simulink model "FMTM"  (R2022b)
settings: Solver=FixedStepAuto  StartTime=0.0  StopTime=10.0  FixedStep=1  RelTol=1e-3
libraries: simulink x34
settings Model: Creator=sadamu  LastModifiedBy=yuzehong
settings OptimizationCC: DefaultParameterBehavior=Inlined  BufferReuse=off  GlobalBufferReuse=off  ExpressionFolding=off  EnableMemcpy=off  PassReuseOutputArgsAs=Individual arguments  NoFixptDivByZeroProtection=on  EfficientFloat2IntCast=on  OptimizeDataStoreBuffers=off  BusAssignmentInplaceUpdate=off  OptimizationLevel=level0  EfficientTunableParamExpr=on
settings DebuggingCC: ParameterTunabilityLossMsg=error  AllowSymbolicDim=off
settings SFSimCC: MATLABDynamicMemAlloc=off
settings RTWCC: Description=Embedded Coder  SystemTargetFile=ert.tlc  GenCodeOnly=on  TemplateMakefile=ert_default_tmf
settings CodeAppCC: GenerateComments=off  IgnoreCustomStorageClasses=off  OperatorAnnotations=on  SimulinkDataObjDesc=on  SFDataObjDesc=on  SimulinkBlockComments=off
settings ERTTargetCC: TargetLangStandard=C99 (ISO)  GenerateSampleERTMain=on  CodeInterfacePackaging=Reusable function  InlinedParameterPlacement=NonHierarchical  ERTCustomFileTemplate=example_file_process.tlc
settings ConfigComp: CovMetricSettings=dcmwe  DVMaxProcessTime=3600  DVTestSuiteOptimization=Auto  DVDetectOutOfBounds=on  DVModelReferenceHarness=on

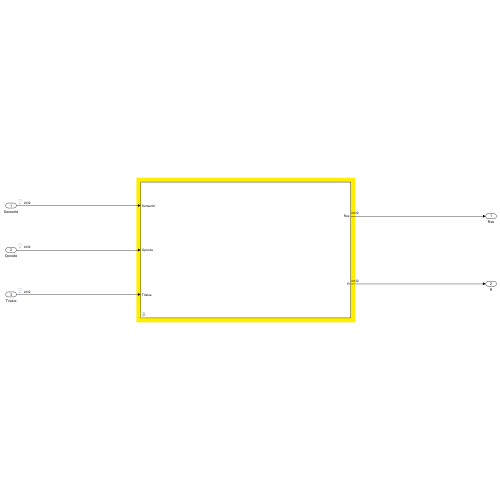
[thumbnail: Simulink's stored preview of the top-level diagram]
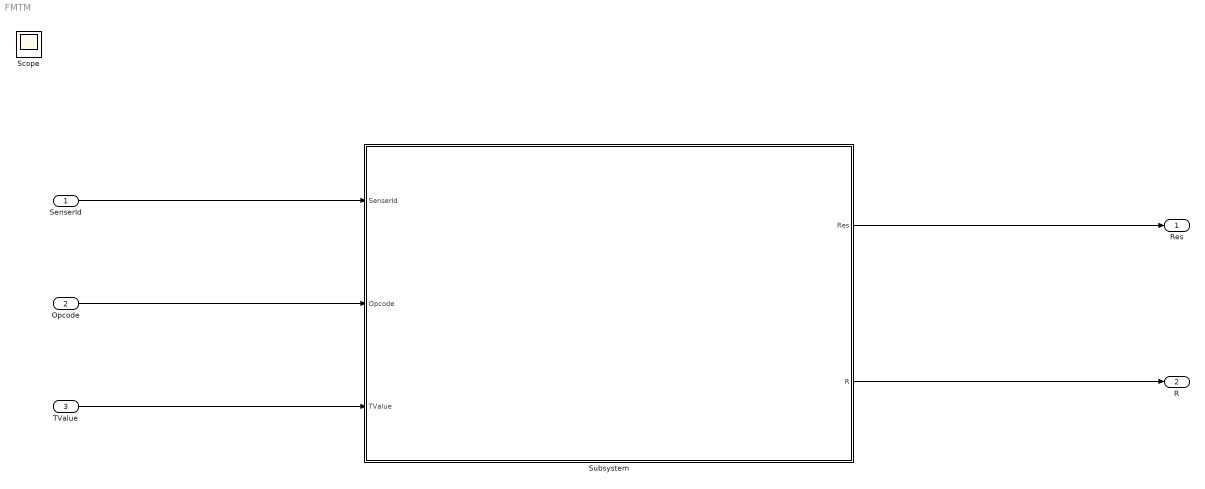
== system FMTM ==
  SenserId : Inport  OutDataTypeStr=int32
  Opcode : Inport  Port=2  OutDataTypeStr=int32
  TValue : Inport  Port=3  OutDataTypeStr=int32
  Subsystem : Subsystem  mask{POOL_SIZE=256}
      mask DialogControl ParameterGroupVar Prompt: 参数
  Res : Outport
  R : Outport  Port=2
  Scope : Scope
  wires:
  SenserId/1 -> Subsystem/1(SenserId)
  Opcode/1 -> Subsystem/2(Opcode)
  TValue/1 -> Subsystem/3(TValue)
  Subsystem/1(Res) -> Res/1
  Subsystem/2(R) -> R/1

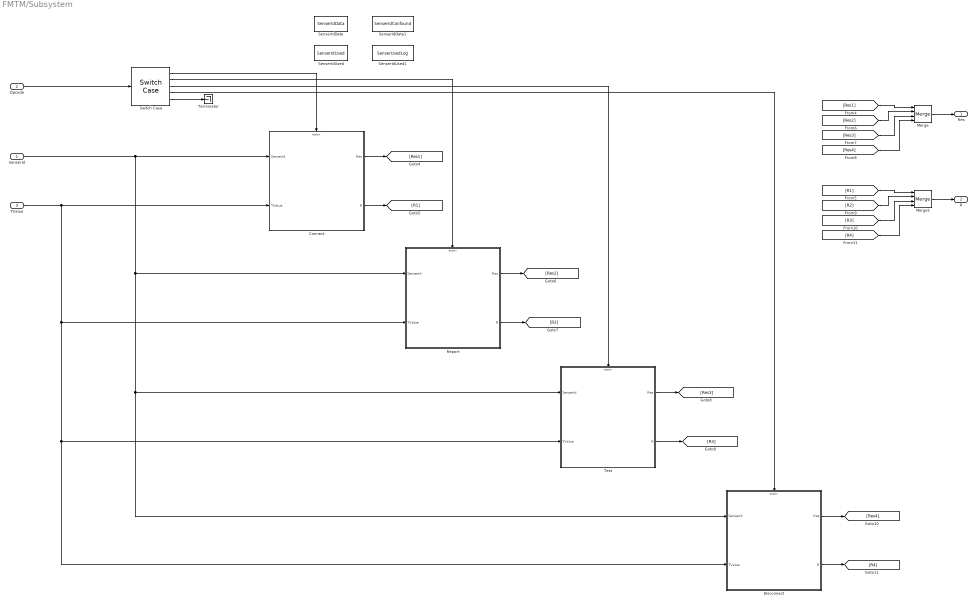
== system FMTM/Subsystem ==
  SenserId : Inport
  Opcode : Inport  Port=2
  TValue : Inport  Port=3
  Connect : Subsystem  TreatAsAtomicUnit=on
  Disconnect : Subsystem  TreatAsAtomicUnit=on
  Merge : Merge  Inputs=4
  Merge1 : Merge  Inputs=4
  Report : Subsystem  TreatAsAtomicUnit=on
  SenserIdData : DataStoreMemory  DataStoreName=SenserIdData  WriteAfterWriteMsg=warning  ShowAdditionalParam=off  OutDataTypeStr=int32  Dimensions=POOL_SIZE
  SenserIdData1 : DataStoreMemory  DataStoreName=SenserIdConfound  WriteAfterWriteMsg=warning  ShowAdditionalParam=off  OutDataTypeStr=int32  Dimensions=POOL_SIZE
  SenserIdUsed : DataStoreMemory  DataStoreName=SenserIdUsed  WriteAfterWriteMsg=warning  ShowAdditionalParam=off  OutDataTypeStr=int32  Dimensions=POOL_SIZE
  SenserIdUsed1 : DataStoreMemory  DataStoreName=SenserUsedLog  WriteAfterWriteMsg=warning  ShowAdditionalParam=off  OutDataTypeStr=int32  Dimensions=POOL_SIZE
  Switch Case : SwitchCase  CaseConditions={1, 3, 4, 5}
  Terminator : Terminator
  Test : Subsystem  TreatAsAtomicUnit=on
  Res : Outport
  R : Outport  Port=2
  wires:
  Connect/1(Res) -> [Res1]
  Opcode/1 -> Switch Case/1
  Test/1(Res) -> [Res3]
  [R4] -> Merge1/4
  [Res1] -> Merge/1
  [R1] -> Merge1/1
  Disconnect/2(R) -> [R4]
  Test/2(R) -> [R3]
  Connect/2(R) -> [R1]
  [Res3] -> Merge/3
  [Res2] -> Merge/2
  [Res4] -> Merge/4
  [R2] -> Merge1/2
  Report/1(Res) -> [Res2]
  [R3] -> Merge1/3
  Switch Case/2 -> Report/Action
  Report/2(R) -> [R2]
  Switch Case/4 -> Disconnect/Action
  SenserId/1 -> Connect/1(SenserId), Test/1(SenserId), Disconnect/1(SenserId), Report/1(SenserId)
  Switch Case/3 -> Test/Action
  TValue/1 -> Connect/2(TValue), Report/2(TValue), Test/2(TValue), Disconnect/2(TValue)
  Disconnect/1(Res) -> [Res4]
  Switch Case/1 -> Connect/Action
  Merge1/1 -> R/1
  Merge/1 -> Res/1
  Switch Case/5 -> Terminator/1

== system FMTM/Subsystem/Connect ==
  SenserId : Inport
  TValue : Inport  Port=2
  Action Port : ActionPort  ActionPortLabel=case [ 1 ]:
  Compare To Constant : simulink/Logic and Bit Operations/Compare To Constant  relop===  const=0  OutDataTypeStr=boolean
  Error : Subsystem  TreatAsAtomicUnit=on
  Handle : Subsystem  TreatAsAtomicUnit=on
  If : If  IfExpression=u1 ~= 0
  Merge : Merge
  Merge1 : Merge
  Res : Outport
  R : Outport  Port=2
  wires:
  SenserId/1 -> Handle/1(SenserId), Compare To Constant/1
  Compare To Constant/1 -> If/1
  If/1 -> Error/Action
  If/2 -> Handle/Action
  Error/1(Res) -> Merge/1
  Handle/1(Res) -> Merge/2
  Merge/1 -> Res/1
  Merge1/1 -> R/1
  Error/2(R) -> Merge1/1
  Handle/2(R) -> Merge1/2
  TValue/1 -> Handle/2(TValue)

== system FMTM/Subsystem/Disconnect ==
  SenserId : Inport
  TValue : Inport  Port=2
  Action Port : ActionPort  ActionPortLabel=case [ 5 ]:
  Compare To Constant : simulink/Logic and Bit Operations/Compare To Constant  relop===  const=0  OutDataTypeStr=boolean
  Error : Subsystem  TreatAsAtomicUnit=on
  Handle : Subsystem  TreatAsAtomicUnit=on
  If : If  IfExpression=u1 ~= 0
  Merge : Merge
  Merge1 : Merge
  Res : Outport
  R : Outport  Port=2
  wires:
  SenserId/1 -> Handle/1(SenserId), Compare To Constant/1
  Compare To Constant/1 -> If/1
  Error/2(R) -> Merge1/1
  TValue/1 -> Handle/2(TValue)
  Handle/1(Res) -> Merge/2
  Merge1/1 -> R/1
  Error/1(Res) -> Merge/1
  Merge/1 -> Res/1
  If/1 -> Error/Action
  If/2 -> Handle/Action
  Handle/2(R) -> Merge1/2

== system FMTM/Subsystem/Report ==
  SenserId : Inport
  TValue : Inport  Port=2
  Action Port : ActionPort  ActionPortLabel=case [ 3 ]:
  Compare To Constant : simulink/Logic and Bit Operations/Compare To Constant  relop===  const=0  OutDataTypeStr=boolean
  Error : Subsystem  TreatAsAtomicUnit=on
  Handle : Subsystem  TreatAsAtomicUnit=on
  If : If  IfExpression=u1 ~= 0
  Merge : Merge
  Merge1 : Merge
  Res : Outport
  R : Outport  Port=2
  wires:
  TValue/1 -> Handle/2(TValue)
  Merge/1 -> Res/1
  Error/2(R) -> Merge1/1
  If/1 -> Error/Action
  If/2 -> Handle/Action
  Merge1/1 -> R/1
  SenserId/1 -> Handle/1(SenserId), Compare To Constant/1
  Error/1(Res) -> Merge/1
  Handle/2(R) -> Merge1/2
  Handle/1(Res) -> Merge/2
  Compare To Constant/1 -> If/1

== system FMTM/Subsystem/Test ==
  SenserId : Inport
  TValue : Inport  Port=2
  Action Port : ActionPort  ActionPortLabel=case [ 4 ]:
  Compare To Constant : simulink/Logic and Bit Operations/Compare To Constant  relop===  const=0  OutDataTypeStr=boolean
  Error : Subsystem  TreatAsAtomicUnit=on
  Handle : Subsystem  TreatAsAtomicUnit=on
  If : If  IfExpression=u1 ~= 0
  Merge : Merge
  Merge1 : Merge
  Res : Outport
  R : Outport  Port=2
  wires:
  TValue/1 -> Handle/2(TValue)
  Merge/1 -> Res/1
  Error/2(R) -> Merge1/1
  If/1 -> Error/Action
  If/2 -> Handle/Action
  Merge1/1 -> R/1
  SenserId/1 -> Handle/1(SenserId), Compare To Constant/1
  Error/1(Res) -> Merge/1
  Handle/2(R) -> Merge1/2
  Handle/1(Res) -> Merge/2
  Compare To Constant/1 -> If/1

== system FMTM/Subsystem/Connect/Error ==
  Action Port : ActionPort  ActionPortLabel=if(u1 ~= 0)
  Constant : Constant  Value=-2  OutDataTypeStr=int32
  Constant1 : Constant  Value=0  OutDataTypeStr=int32
  Res : Outport
  R : Outport  Port=2
  wires:
  Constant/1 -> Res/1
  Constant1/1 -> R/1

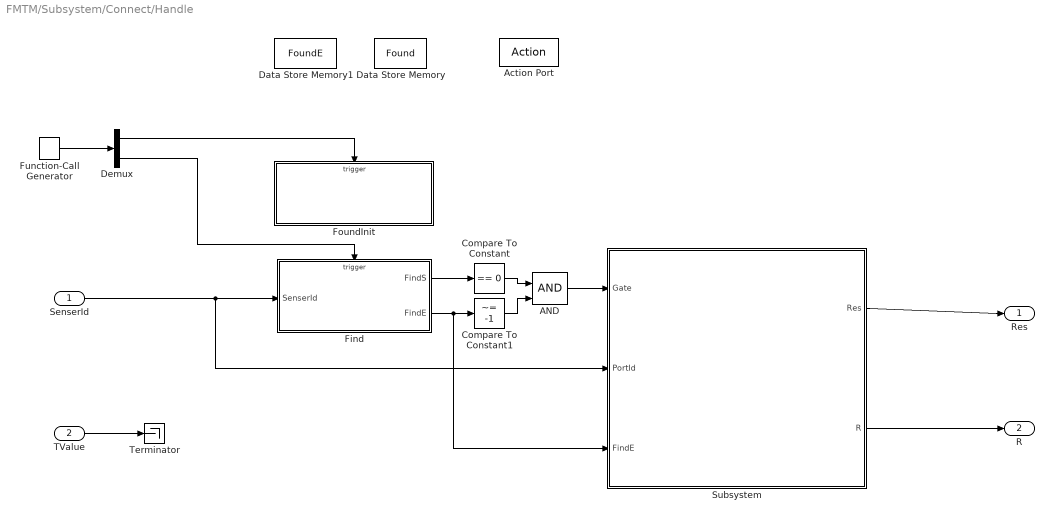
== system FMTM/Subsystem/Connect/Handle ==
  SenserId : Inport
  TValue : Inport  Port=2
  Action Port : ActionPort  ActionPortLabel=else
  AND : Logic  IconShape=distinctive  AllPortsSameDT=off  OutDataTypeStr=boolean
  Compare To Constant : simulink/Logic and Bit Operations/Compare To Constant  relop===  const=0  OutDataTypeStr=boolean
  Compare To Constant1 : simulink/Logic and Bit Operations/Compare To Constant  relop=~=  const=-1  OutDataTypeStr=boolean
  Data Store Memory : DataStoreMemory  DataStoreName=Found  WriteAfterWriteMsg=warning  ShowAdditionalParam=off  OutDataTypeStr=boolean
  Data Store Memory1 : DataStoreMemory  DataStoreName=FoundE  WriteAfterWriteMsg=warning  InitialValue=-1  ShowAdditionalParam=off  OutDataTypeStr=int32
  Demux : Demux  Outputs=2
  Find : Subsystem
  FoundInit : Subsystem
  Function-Call Generator : simulink/Ports & Subsystems/Function-Call Generator  sample_time=1  numberOfIterations=1  DisallowWideOutput=off
  Subsystem : Subsystem
  Terminator : Terminator
  Res : Outport
  R : Outport  Port=2
  wires:
  Function-Call Generator/1 -> Demux/1
  Demux/1 -> FoundInit/Trigger
  Demux/2 -> Find/Trigger
  SenserId/1 -> Subsystem/2(PortId), Find/1(SenserId)
  TValue/1 -> Terminator/1
  Find/1(FindS) -> Compare To Constant/1
  Find/2(FindE) -> Subsystem/3(FindE), Compare To Constant1/1
  Compare To Constant/1 -> AND/1
  Compare To Constant1/1 -> AND/2
  AND/1 -> Subsystem/1(Gate)
  Subsystem/1(Res) -> Res/1
  Subsystem/2(R) -> R/1

== system FMTM/Subsystem/Disconnect/Error ==
  Action Port : ActionPort  ActionPortLabel=if(u1 ~= 0)
  Constant : Constant  Value=-2  OutDataTypeStr=int32
  Constant1 : Constant  Value=0  OutDataTypeStr=int32
  Res : Outport
  R : Outport  Port=2
  wires:
  Constant/1 -> Res/1
  Constant1/1 -> R/1

== system FMTM/Subsystem/Disconnect/Handle ==
  SenserId : Inport
  TValue : Inport  Port=2
  Action Port : ActionPort  ActionPortLabel=else
  Data Store Memory1 : DataStoreMemory  DataStoreName=FoundId  WriteAfterWriteMsg=warning  InitialValue=-1  ShowAdditionalParam=off  OutDataTypeStr=int32
  Demux : Demux  Outputs=2
  Find : Subsystem
  FoundInit : Subsystem
  Function-Call Generator : simulink/Ports & Subsystems/Function-Call Generator  sample_time=1  numberOfIterations=1  DisallowWideOutput=off
  Terminator : Terminator
  Res : Outport
  R : Outport  Port=2
  wires:
  Function-Call Generator/1 -> Demux/1
  Demux/1 -> FoundInit/Trigger
  Demux/2 -> Find/Trigger
  SenserId/1 -> Find/1(SenserId)
  TValue/1 -> Terminator/1
  Find/1(Res) -> Res/1
  Find/2(R) -> R/1

== system FMTM/Subsystem/Report/Error ==
  Action Port : ActionPort  ActionPortLabel=if(u1 ~= 0)
  Constant : Constant  Value=-2  OutDataTypeStr=int32
  Constant1 : Constant  Value=0  OutDataTypeStr=int32
  Res : Outport
  R : Outport  Port=2
  wires:
  Constant/1 -> Res/1
  Constant1/1 -> R/1

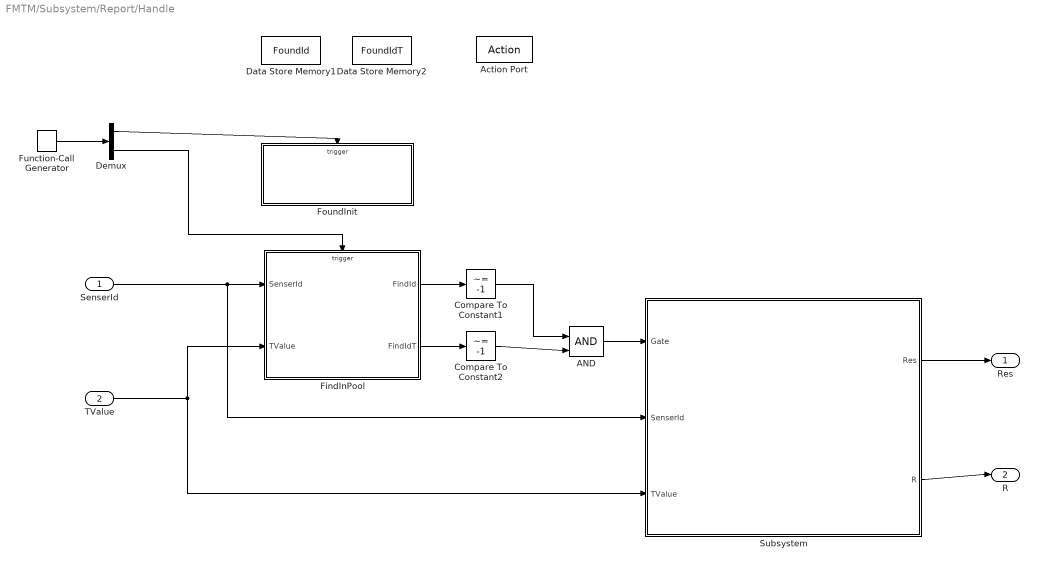
== system FMTM/Subsystem/Report/Handle ==
  SenserId : Inport
  TValue : Inport  Port=2
  Action Port : ActionPort  ActionPortLabel=else
  AND : Logic  IconShape=distinctive  AllPortsSameDT=off  OutDataTypeStr=boolean
  Compare To Constant1 : simulink/Logic and Bit Operations/Compare To Constant  relop=~=  const=-1  OutDataTypeStr=boolean
  Compare To Constant2 : simulink/Logic and Bit Operations/Compare To Constant  relop=~=  const=-1  OutDataTypeStr=boolean
  Data Store Memory1 : DataStoreMemory  DataStoreName=FoundId  WriteAfterWriteMsg=warning  InitialValue=-1  ShowAdditionalParam=off  OutDataTypeStr=int32
  Data Store Memory2 : DataStoreMemory  DataStoreName=FoundIdT  WriteAfterWriteMsg=warning  InitialValue=-1  ShowAdditionalParam=off  OutDataTypeStr=int32
  Demux : Demux  Outputs=2
  FindInPool : Subsystem
  FoundInit : Subsystem
  Function-Call Generator : simulink/Ports & Subsystems/Function-Call Generator  sample_time=1  numberOfIterations=1  DisallowWideOutput=off
  Subsystem : Subsystem
  Res : Outport
  R : Outport  Port=2
  wires:
  Function-Call Generator/1 -> Demux/1
  Demux/1 -> FoundInit/Trigger
  Demux/2 -> FindInPool/Trigger
  SenserId/1 -> Subsystem/2(SenserId), FindInPool/1(SenserId)
  FindInPool/1(FindId) -> Compare To Constant1/1
  TValue/1 -> Subsystem/3(TValue), FindInPool/2(TValue)
  FindInPool/2(FindIdT) -> Compare To Constant2/1
  Compare To Constant1/1 -> AND/1
  Compare To Constant2/1 -> AND/2
  AND/1 -> Subsystem/1(Gate)
  Subsystem/1(Res) -> Res/1
  Subsystem/2(R) -> R/1

== system FMTM/Subsystem/Test/Error ==
  Action Port : ActionPort  ActionPortLabel=if(u1 ~= 0)
  Constant : Constant  Value=-2  OutDataTypeStr=int32
  Constant1 : Constant  Value=0  OutDataTypeStr=int32
  Res : Outport
  R : Outport  Port=2
  wires:
  Constant/1 -> Res/1
  Constant1/1 -> R/1

== system FMTM/Subsystem/Test/Handle ==
  SenserId : Inport
  TValue : Inport  Port=2
  Action Port : ActionPort  ActionPortLabel=else
  Compare To Constant : simulink/Logic and Bit Operations/Compare To Constant  relop=~=  const=-1  OutDataTypeStr=boolean
  Data Store Memory1 : DataStoreMemory  DataStoreName=FoundId  WriteAfterWriteMsg=warning  InitialValue=-1  ShowAdditionalParam=off  OutDataTypeStr=int32
  Demux : Demux  Outputs=2
  FindInPool : Subsystem
  FoundInit : Subsystem
  Function-Call Generator : simulink/Ports & Subsystems/Function-Call Generator  sample_time=1  numberOfIterations=1  DisallowWideOutput=off
  Subsystem : Subsystem
  Terminator : Terminator
  Res : Outport
  R : Outport  Port=2
  wires:
  Function-Call Generator/1 -> Demux/1
  Demux/1 -> FoundInit/Trigger
  Demux/2 -> FindInPool/Trigger
  SenserId/1 -> FindInPool/1(SenserId)
  TValue/1 -> Terminator/1
  FindInPool/1(FindId) -> Subsystem/1(FindId), Compare To Constant/1
  Compare To Constant/1 -> Subsystem/2(Gate)
  Subsystem/1(Res) -> Res/1
  Subsystem/2(R) -> R/1

== system FMTM/Subsystem/Connect/Handle/Find ==
  SenserId : Inport
  function : TriggerPort  TriggerType=function-call  VariantControl=(inherit)
  FindEmpty : Subsystem  TreatAsAtomicUnit=on
  FindSenserId : Subsystem  TreatAsAtomicUnit=on
  FindS : Outport
  FindE : Outport  Port=2
  wires:
  FindSenserId/1(Out1) -> FindS/1
  SenserId/1 -> FindSenserId/1(SenserId)
  FindEmpty/1(Out1) -> FindE/1

== system FMTM/Subsystem/Connect/Handle/FoundInit ==
  function : TriggerPort  TriggerType=function-call  VariantControl=(inherit)
  Constant : Constant  Value=0  OutDataTypeStr=boolean
  Constant1 : Constant  Value=-1  OutDataTypeStr=int32
  Data Store Write : DataStoreWrite  DataStoreName=Found  IndexOptions=Index vector (dialog)  Indices=1  OutputSizes=1
  Data Store Write1 : DataStoreWrite  DataStoreName=FoundE  IndexOptions=Index vector (dialog)  Indices=1  OutputSizes=1
  wires:
  Constant/1 -> Data Store Write/1
  Constant1/1 -> Data Store Write1/1

== system FMTM/Subsystem/Connect/Handle/Subsystem ==
  Gate : Inport
  PortId : Inport  Port=2
  FindE : Inport  Port=3
  AddSenserId : Subsystem  TreatAsAtomicUnit=on
  Err : Subsystem  TreatAsAtomicUnit=on
  If : If  IfExpression=u1 ~= 0
  Merge : Merge
  Res : Outport
  R : Outport  Port=2
  wires:
  Merge/1 -> Res/1
  If/2 -> Err/Action
  If/1 -> AddSenserId/Action
  AddSenserId/2(R) -> R/1
  AddSenserId/1(Res) -> Merge/2
  PortId/1 -> AddSenserId/1(PortId)
  Err/1(Result) -> Merge/1
  Gate/1 -> If/1
  FindE/1 -> AddSenserId/2(FindE)

== system FMTM/Subsystem/Disconnect/Handle/Find ==
  SenserId : Inport
  function : TriggerPort  TriggerType=function-call  VariantControl=(inherit)
  Compare To Constant1 : simulink/Logic and Bit Operations/Compare To Constant  relop===  const=-1  OutDataTypeStr=uint8
  FindSenserId : Subsystem  TreatAsAtomicUnit=on
  Subsystem : Subsystem
  Res : Outport
  R : Outport  Port=2
  wires:
  SenserId/1 -> Subsystem/1(SenserId), FindSenserId/1(SenserId)
  FindSenserId/1(Out1) -> Compare To Constant1/1
  Compare To Constant1/1 -> Subsystem/2(Gate)
  Subsystem/1(Out1) -> Res/1
  Subsystem/2(Out2) -> R/1

== system FMTM/Subsystem/Disconnect/Handle/FoundInit ==
  function : TriggerPort  TriggerType=function-call  VariantControl=(inherit)
  Constant1 : Constant  Value=-1  OutDataTypeStr=int32
  Data Store Write1 : DataStoreWrite  DataStoreName=FoundId  IndexOptions=Index vector (dialog)  Indices=1  OutputSizes=1
  wires:
  Constant1/1 -> Data Store Write1/1

== system FMTM/Subsystem/Report/Handle/FindInPool ==
  SenserId : Inport
  TValue : Inport  Port=2
  function : TriggerPort  TriggerType=function-call  VariantControl=(inherit)
  FindSenserId : Subsystem  TreatAsAtomicUnit=on
  FindSenserIdT : Subsystem  TreatAsAtomicUnit=on
  FindId : Outport
  FindIdT : Outport  Port=2
  wires:
  SenserId/1 -> FindSenserId/1(SenserId)
  FindSenserId/1(Out1) -> FindId/1
  TValue/1 -> FindSenserIdT/1(TValue)
  FindSenserIdT/1(FindPT) -> FindIdT/1

== system FMTM/Subsystem/Report/Handle/FoundInit ==
  function : TriggerPort  TriggerType=function-call  VariantControl=(inherit)
  Constant1 : Constant  Value=-1  OutDataTypeStr=int32
  Constant2 : Constant  Value=-1  OutDataTypeStr=int32
  Data Store Write1 : DataStoreWrite  DataStoreName=FoundId  IndexOptions=Index vector (dialog)  Indices=1  OutputSizes=1
  Data Store Write2 : DataStoreWrite  DataStoreName=FoundIdT  IndexOptions=Index vector (dialog)  Indices=1  OutputSizes=1
  wires:
  Constant1/1 -> Data Store Write1/1
  Constant2/1 -> Data Store Write2/1

== system FMTM/Subsystem/Report/Handle/Subsystem ==
  Gate : Inport
  SenserId : Inport  Port=2
  TValue : Inport  Port=3
  Err : Subsystem  TreatAsAtomicUnit=on
  If : If  IfExpression=u1 ~= 0
  Merge : Merge
  SetSenserId : Subsystem  TreatAsAtomicUnit=on
  Res : Outport
  R : Outport  Port=2
  wires:
  If/1 -> SetSenserId/Action
  SetSenserId/1(Res) -> Merge/2
  TValue/1 -> SetSenserId/2(TValue)
  Gate/1 -> If/1
  Err/1(Res) -> Merge/1
  If/2 -> Err/Action
  Merge/1 -> Res/1
  SetSenserId/2(R) -> R/1
  SenserId/1 -> SetSenserId/1(SenserId)

== system FMTM/Subsystem/Test/Handle/FindInPool ==
  SenserId : Inport
  function : TriggerPort  TriggerType=function-call  VariantControl=(inherit)
  FindSenserId : Subsystem  TreatAsAtomicUnit=on
  FindId : Outport
  wires:
  SenserId/1 -> FindSenserId/1(SenserId)
  FindSenserId/1(FindId) -> FindId/1

== system FMTM/Subsystem/Test/Handle/FoundInit ==
  function : TriggerPort  TriggerType=function-call  VariantControl=(inherit)
  Constant1 : Constant  Value=-1  OutDataTypeStr=int32
  Data Store Write1 : DataStoreWrite  DataStoreName=FoundId  IndexOptions=Index vector (dialog)  Indices=1  OutputSizes=1
  wires:
  Constant1/1 -> Data Store Write1/1

== system FMTM/Subsystem/Test/Handle/Subsystem ==
  FindId : Inport
  Gate : Inport  Port=2
  If : If  IfExpression=u1 ~= 0
  If Action Subsystem : Subsystem  TreatAsAtomicUnit=on
  If Action Subsystem1 : Subsystem  TreatAsAtomicUnit=on
  Merge : Merge
  Merge1 : Merge
  Res : Outport
  R : Outport  Port=2
  wires:
  If Action Subsystem/2(R) -> Merge1/1
  If/2 -> If Action Subsystem1/Action
  If Action Subsystem1/1(Res) -> Merge/2
  If/1 -> If Action Subsystem/Action
  If Action Subsystem1/2(R) -> Merge1/2
  Merge1/1 -> R/1
  If Action Subsystem/1(Res) -> Merge/1
  Gate/1 -> If/1
  Merge/1 -> Res/1
  FindId/1 -> If Action Subsystem/1(FindId)

== system FMTM/Subsystem/Connect/Handle/Find/FindEmpty ==
  AND : Logic  IconShape=distinctive  AllPortsSameDT=off  OutDataTypeStr=boolean
  Compare To Constant1 : simulink/Logic and Bit Operations/Compare To Constant  relop===  const=-1  OutDataTypeStr=boolean
  Compare To Constant2 : simulink/Logic and Bit Operations/Compare To Constant  relop===  const=0  OutDataTypeStr=boolean
  Data Store Read1 : DataStoreRead  DataStoreName=FoundE  IndexOptions=Index vector (dialog)  Indices=1  OutputSizes=1
  Data Store Read2 : DataStoreRead  DataStoreName=SenserIdUsed  IndexOptions=Index vector (dialog)  Indices=1  OutputSizes=1
  Data Store Write1 : DataStoreWrite  DataStoreName=FoundE  IndexOptions=Index vector (dialog)  Indices=1  OutputSizes=1
  For Iterator : ForIterator  IterationLimit=POOL_SIZE  IndexMode=Zero-based
  Selector1 : Selector  IndexMode=Zero-based  InputPortWidth=POOL_SIZE  IndexOptions=Index vector (port)  Indices=[1 3]  OutputSizes=1
  Switch : Switch  Criteria=u2 ~= 0  SaturateOnIntegerOverflow=off  InputSameDT=off
  Out1 : Outport
  wires:
  Switch/1 -> Data Store Write1/1, Out1/1
  Data Store Read1/1 -> Compare To Constant1/1, Switch/3
  Compare To Constant1/1 -> AND/2
  AND/1 -> Switch/2
  For Iterator/1 -> Selector1/2, Switch/1
  Selector1/1 -> Compare To Constant2/1
  Data Store Read2/1 -> Selector1/1
  Compare To Constant2/1 -> AND/1

== system FMTM/Subsystem/Connect/Handle/Find/FindSenserId ==
  SenserId : Inport
  AND : Logic  IconShape=distinctive  AllPortsSameDT=off  OutDataTypeStr=boolean
  Compare To Constant : simulink/Logic and Bit Operations/Compare To Constant  relop===  const=1  OutDataTypeStr=boolean
  Constant : Constant  OutDataTypeStr=boolean
  Data Store Read : DataStoreRead  DataStoreName=SenserIdUsed  IndexOptions=Index vector (dialog)  Indices=1  OutputSizes=1
  Data Store Read1 : DataStoreRead  DataStoreName=Found  IndexOptions=Index vector (dialog)  Indices=1  OutputSizes=1
  Data Store Read2 : DataStoreRead  DataStoreName=SenserIdUsed  IndexOptions=Index vector (dialog)  Indices=1  OutputSizes=1
  Data Store Write1 : DataStoreWrite  DataStoreName=Found  IndexOptions=Index vector (dialog)  Indices=1  OutputSizes=1
  Equal : RelationalOperator  Operator===  OutDataTypeStr=boolean  RndMeth=Simplest  InputSameDT=off
  For Iterator : ForIterator  IterationLimit=POOL_SIZE  IndexMode=Zero-based
  Selector : Selector  IndexMode=Zero-based  InputPortWidth=POOL_SIZE  IndexOptions=Index vector (port)  Indices=[1 3]  OutputSizes=1
  Selector1 : Selector  IndexMode=Zero-based  InputPortWidth=POOL_SIZE  IndexOptions=Index vector (port)  Indices=[1 3]  OutputSizes=1
  Switch : Switch  Criteria=u2 ~= 0  SaturateOnIntegerOverflow=off  InputSameDT=off
  Out1 : Outport
  wires:
  For Iterator/1 -> Selector1/2, Selector/2
  Data Store Read/1 -> Selector/1
  Selector/1 -> Equal/1
  SenserId/1 -> Equal/2
  Equal/1 -> AND/1
  Constant/1 -> Switch/1
  Switch/1 -> Out1/1, Data Store Write1/1
  Data Store Read1/1 -> Switch/3
  Data Store Read2/1 -> Selector1/1
  Selector1/1 -> Compare To Constant/1
  Compare To Constant/1 -> AND/2
  AND/1 -> Switch/2

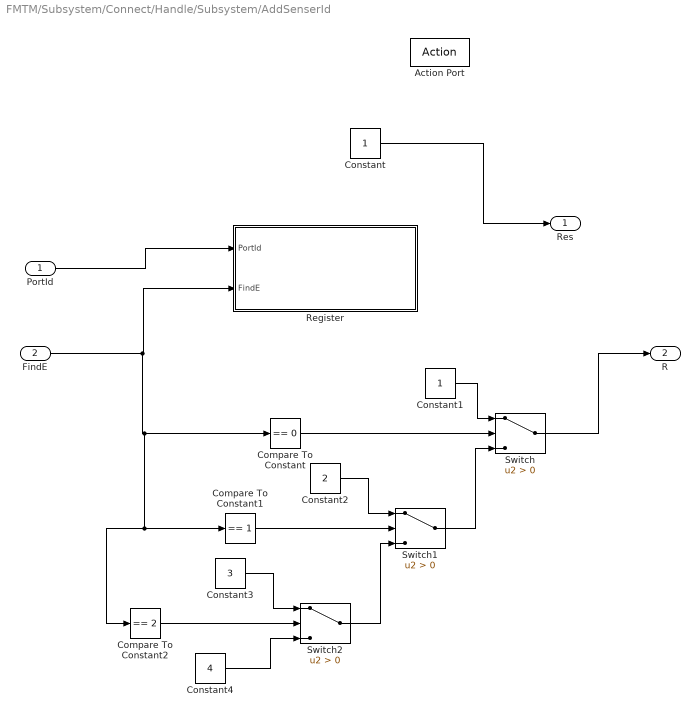
== system FMTM/Subsystem/Connect/Handle/Subsystem/AddSenserId ==
  PortId : Inport
  FindE : Inport  Port=2
  Action Port : ActionPort  ActionPortLabel=if(u1 ~= 0)
  Compare To Constant : simulink/Logic and Bit Operations/Compare To Constant  relop===  const=0  OutDataTypeStr=boolean
  Compare To Constant1 : simulink/Logic and Bit Operations/Compare To Constant  relop===  const=1  OutDataTypeStr=boolean
  Compare To Constant2 : simulink/Logic and Bit Operations/Compare To Constant  relop===  const=2  OutDataTypeStr=boolean
  Constant : Constant  OutDataTypeStr=int32
  Constant1 : Constant  OutDataTypeStr=int32
  Constant2 : Constant  Value=2  OutDataTypeStr=int32
  Constant3 : Constant  Value=3  OutDataTypeStr=int32
  Constant4 : Constant  Value=4  OutDataTypeStr=int32
  Register : Subsystem  TreatAsAtomicUnit=on
  Switch : Switch  Criteria=u2 > Threshold  SaturateOnIntegerOverflow=off  InputSameDT=off
  Switch1 : Switch  Criteria=u2 > Threshold  SaturateOnIntegerOverflow=off  InputSameDT=off
  Switch2 : Switch  Criteria=u2 > Threshold  SaturateOnIntegerOverflow=off  InputSameDT=off
  Res : Outport
  R : Outport  Port=2
  wires:
  PortId/1 -> Register/1(PortId)
  FindE/1 -> Compare To Constant2/1, Compare To Constant1/1, Compare To Constant/1, Register/2(FindE)
  Constant/1 -> Res/1
  Compare To Constant/1 -> Switch/2
  Constant1/1 -> Switch/1
  Constant2/1 -> Switch1/1
  Compare To Constant1/1 -> Switch1/2
  Switch1/1 -> Switch/3
  Compare To Constant2/1 -> Switch2/2
  Switch2/1 -> Switch1/3
  Constant3/1 -> Switch2/1
  Constant4/1 -> Switch2/3
  Switch/1 -> R/1

== system FMTM/Subsystem/Connect/Handle/Subsystem/Err ==
  Action Port : ActionPort  ActionPortLabel=else
  Constant : Constant  Value=-10004  OutDataTypeStr=int32
  Result : Outport
  wires:
  Constant/1 -> Result/1

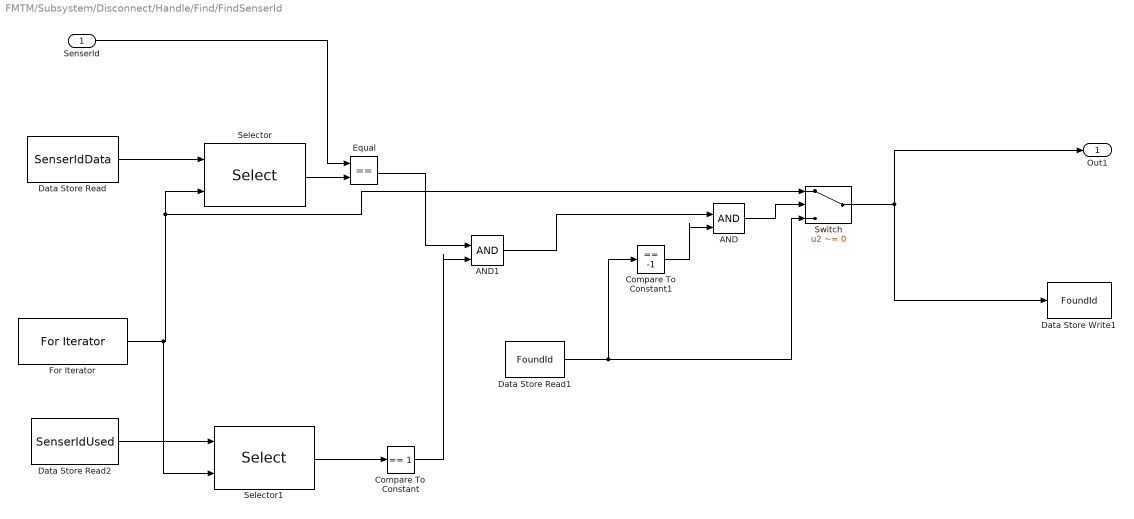
== system FMTM/Subsystem/Disconnect/Handle/Find/FindSenserId ==
  SenserId : Inport
  AND : Logic  IconShape=distinctive  AllPortsSameDT=off  OutDataTypeStr=boolean
  AND1 : Logic  IconShape=distinctive  AllPortsSameDT=off  OutDataTypeStr=boolean
  Compare To Constant : simulink/Logic and Bit Operations/Compare To Constant  relop===  const=1  OutDataTypeStr=boolean
  Compare To Constant1 : simulink/Logic and Bit Operations/Compare To Constant  relop===  const=-1  OutDataTypeStr=boolean
  Data Store Read : DataStoreRead  DataStoreName=SenserIdData  IndexOptions=Index vector (dialog)  Indices=1  OutputSizes=1
  Data Store Read1 : DataStoreRead  DataStoreName=FoundId  IndexOptions=Index vector (dialog)  Indices=1  OutputSizes=1
  Data Store Read2 : DataStoreRead  DataStoreName=SenserIdUsed  IndexOptions=Index vector (dialog)  Indices=1  OutputSizes=1
  Data Store Write1 : DataStoreWrite  DataStoreName=FoundId  IndexOptions=Index vector (dialog)  Indices=1  OutputSizes=1
  Equal : RelationalOperator  Operator===  OutDataTypeStr=boolean  RndMeth=Simplest  InputSameDT=off
  For Iterator : ForIterator  IterationLimit=POOL_SIZE  IndexMode=Zero-based
  Selector : Selector  IndexMode=Zero-based  InputPortWidth=POOL_SIZE  IndexOptions=Index vector (port)  Indices=[1 3]  OutputSizes=1
  Selector1 : Selector  IndexMode=Zero-based  InputPortWidth=POOL_SIZE  IndexOptions=Index vector (port)  Indices=[1 3]  OutputSizes=1
  Switch : Switch  Criteria=u2 ~= 0  SaturateOnIntegerOverflow=off  InputSameDT=off
  Out1 : Outport
  wires:
  Data Store Read/1 -> Selector/1
  Selector/1 -> Equal/2
  Equal/1 -> AND1/1
  Switch/1 -> Data Store Write1/1, Out1/1
  Data Store Read1/1 -> Compare To Constant1/1, Switch/3
  Compare To Constant1/1 -> AND/2
  AND/1 -> Switch/2
  SenserId/1 -> Equal/1
  Compare To Constant/1 -> AND1/2
  Data Store Read2/1 -> Selector1/1
  For Iterator/1 -> Selector1/2, Switch/1, Selector/2
  Selector1/1 -> Compare To Constant/1
  AND1/1 -> AND/1

== system FMTM/Subsystem/Disconnect/Handle/Find/Subsystem ==
  SenserId : Inport
  Gate : Inport  Port=2
  Err : Subsystem  TreatAsAtomicUnit=on
  If : If  IfExpression=u1 ~= 0
  Merge : Merge
  Merge1 : Merge
  SetSenserId : Subsystem  TreatAsAtomicUnit=on
  Out1 : Outport
  Out2 : Outport  Port=2
  wires:
  Merge/1 -> Out1/1
  Merge1/1 -> Out2/1
  If/2 -> SetSenserId/Action
  Err/2(R) -> Merge1/1
  Err/1(Result) -> Merge/1
  SetSenserId/1(Res) -> Merge/2
  SetSenserId/2(R) -> Merge1/2
  If/1 -> Err/Action
  SenserId/1 -> SetSenserId/1(SenserId)
  Gate/1 -> If/1

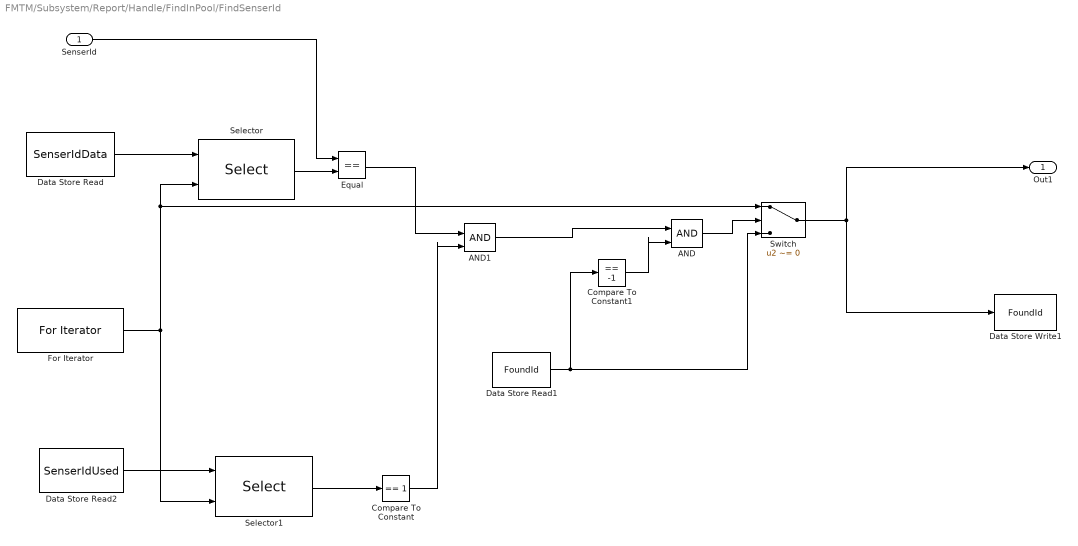
== system FMTM/Subsystem/Report/Handle/FindInPool/FindSenserId ==
  SenserId : Inport
  AND : Logic  IconShape=distinctive  AllPortsSameDT=off  OutDataTypeStr=boolean
  AND1 : Logic  IconShape=distinctive  AllPortsSameDT=off  OutDataTypeStr=boolean
  Compare To Constant : simulink/Logic and Bit Operations/Compare To Constant  relop===  const=1  OutDataTypeStr=boolean
  Compare To Constant1 : simulink/Logic and Bit Operations/Compare To Constant  relop===  const=-1  OutDataTypeStr=boolean
  Data Store Read : DataStoreRead  DataStoreName=SenserIdData  IndexOptions=Index vector (dialog)  Indices=1  OutputSizes=1
  Data Store Read1 : DataStoreRead  DataStoreName=FoundId  IndexOptions=Index vector (dialog)  Indices=1  OutputSizes=1
  Data Store Read2 : DataStoreRead  DataStoreName=SenserIdUsed  IndexOptions=Index vector (dialog)  Indices=1  OutputSizes=1
  Data Store Write1 : DataStoreWrite  DataStoreName=FoundId  IndexOptions=Index vector (dialog)  Indices=1  OutputSizes=1
  Equal : RelationalOperator  Operator===  OutDataTypeStr=boolean  RndMeth=Simplest  InputSameDT=off
  For Iterator : ForIterator  IterationLimit=POOL_SIZE  IndexMode=Zero-based
  Selector : Selector  IndexMode=Zero-based  InputPortWidth=POOL_SIZE  IndexOptions=Index vector (port)  Indices=[1 3]  OutputSizes=1
  Selector1 : Selector  IndexMode=Zero-based  InputPortWidth=POOL_SIZE  IndexOptions=Index vector (port)  Indices=[1 3]  OutputSizes=1
  Switch : Switch  Criteria=u2 ~= 0  SaturateOnIntegerOverflow=off  InputSameDT=off
  Out1 : Outport
  wires:
  Data Store Read/1 -> Selector/1
  Selector/1 -> Equal/2
  Equal/1 -> AND1/1
  Switch/1 -> Data Store Write1/1, Out1/1
  Data Store Read1/1 -> Compare To Constant1/1, Switch/3
  Compare To Constant1/1 -> AND/2
  AND/1 -> Switch/2
  SenserId/1 -> Equal/1
  For Iterator/1 -> Selector1/2, Switch/1, Selector/2
  Selector1/1 -> Compare To Constant/1
  Data Store Read2/1 -> Selector1/1
  Compare To Constant/1 -> AND1/2
  AND1/1 -> AND/1

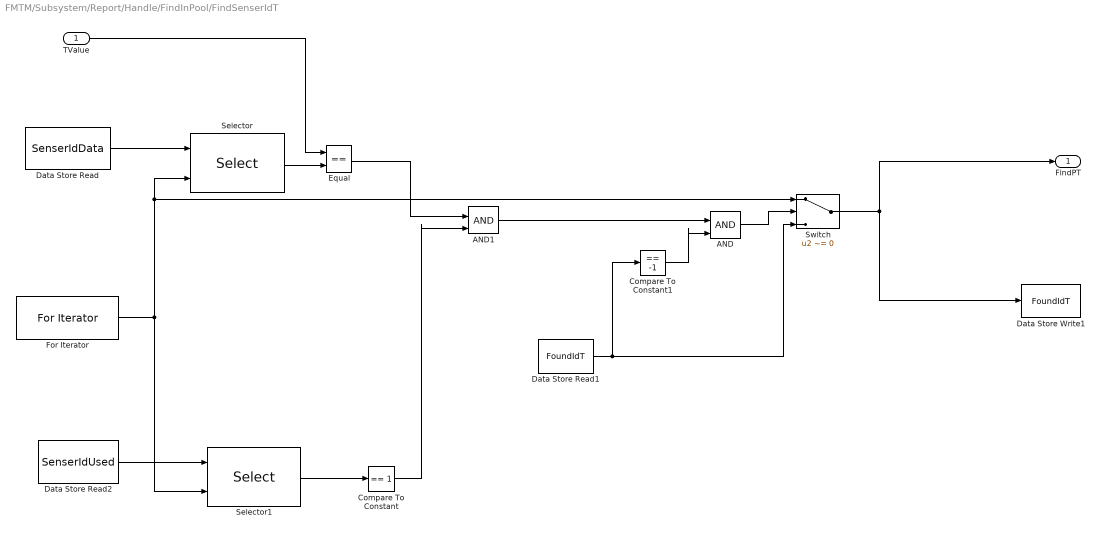
== system FMTM/Subsystem/Report/Handle/FindInPool/FindSenserIdT ==
  TValue : Inport
  AND : Logic  IconShape=distinctive  AllPortsSameDT=off  OutDataTypeStr=boolean
  AND1 : Logic  IconShape=distinctive  AllPortsSameDT=off  OutDataTypeStr=boolean
  Compare To Constant : simulink/Logic and Bit Operations/Compare To Constant  relop===  const=1  OutDataTypeStr=boolean
  Compare To Constant1 : simulink/Logic and Bit Operations/Compare To Constant  relop===  const=-1  OutDataTypeStr=boolean
  Data Store Read : DataStoreRead  DataStoreName=SenserIdData  IndexOptions=Index vector (dialog)  Indices=1  OutputSizes=1
  Data Store Read1 : DataStoreRead  DataStoreName=FoundIdT  IndexOptions=Index vector (dialog)  Indices=1  OutputSizes=1
  Data Store Read2 : DataStoreRead  DataStoreName=SenserIdUsed  IndexOptions=Index vector (dialog)  Indices=1  OutputSizes=1
  Data Store Write1 : DataStoreWrite  DataStoreName=FoundIdT  IndexOptions=Index vector (dialog)  Indices=1  OutputSizes=1
  Equal : RelationalOperator  Operator===  OutDataTypeStr=boolean  RndMeth=Simplest  InputSameDT=off
  For Iterator : ForIterator  IterationLimit=POOL_SIZE  IndexMode=Zero-based
  Selector : Selector  IndexMode=Zero-based  InputPortWidth=POOL_SIZE  IndexOptions=Index vector (port)  Indices=[1 3]  OutputSizes=1
  Selector1 : Selector  IndexMode=Zero-based  InputPortWidth=POOL_SIZE  IndexOptions=Index vector (port)  Indices=[1 3]  OutputSizes=1
  Switch : Switch  Criteria=u2 ~= 0  SaturateOnIntegerOverflow=off  InputSameDT=off
  FindPT : Outport
  wires:
  Data Store Read/1 -> Selector/1
  Selector/1 -> Equal/2
  Equal/1 -> AND1/1
  Switch/1 -> Data Store Write1/1, FindPT/1
  Data Store Read1/1 -> Compare To Constant1/1, Switch/3
  Compare To Constant1/1 -> AND/2
  AND/1 -> Switch/2
  TValue/1 -> Equal/1
  Compare To Constant/1 -> AND1/2
  Data Store Read2/1 -> Selector1/1
  For Iterator/1 -> Selector1/2, Switch/1, Selector/2
  Selector1/1 -> Compare To Constant/1
  AND1/1 -> AND/1

== system FMTM/Subsystem/Report/Handle/Subsystem/Err ==
  Action Port : ActionPort  ActionPortLabel=else
  Constant : Constant  Value=-8  OutDataTypeStr=int32
  Res : Outport
  wires:
  Constant/1 -> Res/1

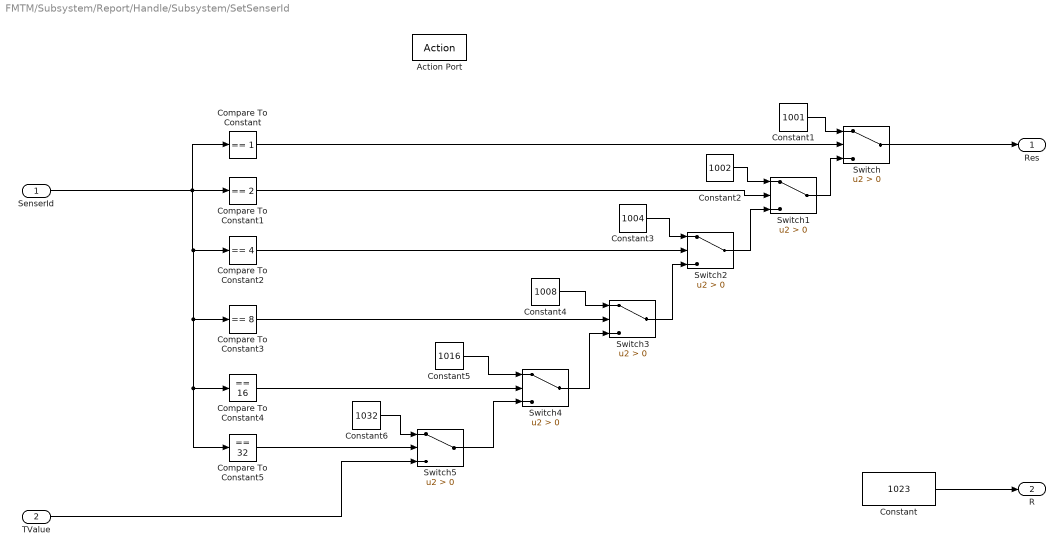
== system FMTM/Subsystem/Report/Handle/Subsystem/SetSenserId ==
  SenserId : Inport
  TValue : Inport  Port=2
  Action Port : ActionPort  ActionPortLabel=if(u1 ~= 0)
  Compare To Constant : simulink/Logic and Bit Operations/Compare To Constant  relop===  const=1  OutDataTypeStr=boolean
  Compare To Constant1 : simulink/Logic and Bit Operations/Compare To Constant  relop===  const=2  OutDataTypeStr=boolean
  Compare To Constant2 : simulink/Logic and Bit Operations/Compare To Constant  relop===  const=4  OutDataTypeStr=boolean
  Compare To Constant3 : simulink/Logic and Bit Operations/Compare To Constant  relop===  const=8  OutDataTypeStr=boolean
  Compare To Constant4 : simulink/Logic and Bit Operations/Compare To Constant  relop===  const=16  OutDataTypeStr=boolean
  Compare To Constant5 : simulink/Logic and Bit Operations/Compare To Constant  relop===  const=32  OutDataTypeStr=boolean
  Constant : Constant  Value=1023  OutDataTypeStr=int32
  Constant1 : Constant  Value=1001  OutDataTypeStr=int32
  Constant2 : Constant  Value=1002  OutDataTypeStr=int32
  Constant3 : Constant  Value=1004  OutDataTypeStr=int32
  Constant4 : Constant  Value=1008  OutDataTypeStr=int32
  Constant5 : Constant  Value=1016  OutDataTypeStr=int32
  Constant6 : Constant  Value=1032  OutDataTypeStr=int32
  Switch{,1..5} (6 alike) : Switch  Criteria=u2 > Threshold  SaturateOnIntegerOverflow=off  InputSameDT=off
  Res : Outport
  R : Outport  Port=2
  wires:
  Constant/1 -> R/1
  Switch2/1 -> Switch1/3
  SenserId/1 -> Compare To Constant5/1, Compare To Constant4/1, Compare To Constant3/1, Compare To Constant2/1, Compare To Constant/1, Compare To Constant1/1
  Switch1/1 -> Switch/3
  Constant3/1 -> Switch2/1
  Compare To Constant2/1 -> Switch2/2
  Constant2/1 -> Switch1/1
  Constant1/1 -> Switch/1
  Switch/1 -> Res/1
  Compare To Constant/1 -> Switch/2
  Compare To Constant1/1 -> Switch1/2
  Switch4/1 -> Switch3/3
  Switch3/1 -> Switch2/3
  Constant6/1 -> Switch5/1
  Compare To Constant3/1 -> Switch3/2
  Constant5/1 -> Switch4/1
  Switch5/1 -> Switch4/3
  Compare To Constant4/1 -> Switch4/2
  Constant4/1 -> Switch3/1
  Compare To Constant5/1 -> Switch5/2
  TValue/1 -> Switch5/3

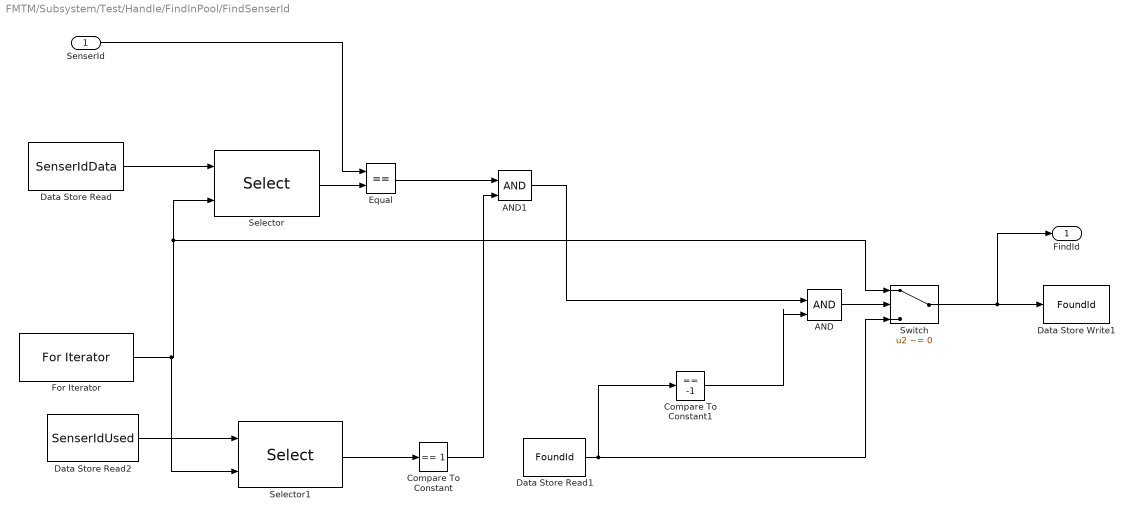
== system FMTM/Subsystem/Test/Handle/FindInPool/FindSenserId ==
  SenserId : Inport
  AND : Logic  IconShape=distinctive  AllPortsSameDT=off  OutDataTypeStr=boolean
  AND1 : Logic  IconShape=distinctive  AllPortsSameDT=off  OutDataTypeStr=boolean
  Compare To Constant : simulink/Logic and Bit Operations/Compare To Constant  relop===  const=1  OutDataTypeStr=boolean
  Compare To Constant1 : simulink/Logic and Bit Operations/Compare To Constant  relop===  const=-1  OutDataTypeStr=boolean
  Data Store Read : DataStoreRead  DataStoreName=SenserIdData  IndexOptions=Index vector (dialog)  Indices=1  OutputSizes=1
  Data Store Read1 : DataStoreRead  DataStoreName=FoundId  IndexOptions=Index vector (dialog)  Indices=1  OutputSizes=1
  Data Store Read2 : DataStoreRead  DataStoreName=SenserIdUsed  IndexOptions=Index vector (dialog)  Indices=1  OutputSizes=1
  Data Store Write1 : DataStoreWrite  DataStoreName=FoundId  IndexOptions=Index vector (dialog)  Indices=1  OutputSizes=1
  Equal : RelationalOperator  Operator===  OutDataTypeStr=boolean  RndMeth=Simplest  InputSameDT=off
  For Iterator : ForIterator  IterationLimit=POOL_SIZE  IndexMode=Zero-based
  Selector : Selector  IndexMode=Zero-based  InputPortWidth=POOL_SIZE  IndexOptions=Index vector (port)  Indices=[1 3]  OutputSizes=1
  Selector1 : Selector  IndexMode=Zero-based  InputPortWidth=POOL_SIZE  IndexOptions=Index vector (port)  Indices=[1 3]  OutputSizes=1
  Switch : Switch  Criteria=u2 ~= 0  SaturateOnIntegerOverflow=off  InputSameDT=off
  FindId : Outport
  wires:
  Data Store Read/1 -> Selector/1
  Selector/1 -> Equal/2
  Equal/1 -> AND1/1
  Switch/1 -> FindId/1, Data Store Write1/1
  Data Store Read1/1 -> Compare To Constant1/1, Switch/3
  Compare To Constant1/1 -> AND/2
  AND/1 -> Switch/2
  SenserId/1 -> Equal/1
  Compare To Constant/1 -> AND1/2
  Data Store Read2/1 -> Selector1/1
  For Iterator/1 -> Selector1/2, Selector/2, Switch/1
  Selector1/1 -> Compare To Constant/1
  AND1/1 -> AND/1

== system FMTM/Subsystem/Test/Handle/Subsystem/If Action Subsystem ==
  FindId : Inport
  Action Port : ActionPort  ActionPortLabel=if(u1 ~= 0)
  Constant : Constant  OutDataTypeStr=int32
  Res : Outport
  R : Outport  Port=2
  wires:
  FindId/1 -> Res/1
  Constant/1 -> R/1

== system FMTM/Subsystem/Test/Handle/Subsystem/If Action Subsystem1 ==
  Action Port : ActionPort  ActionPortLabel=else
  Constant : Constant  Value=-1  OutDataTypeStr=int32
  Constant1 : Constant  Value=-1  OutDataTypeStr=int32
  Res : Outport
  R : Outport  Port=2
  wires:
  Constant/1 -> R/1
  Constant1/1 -> Res/1

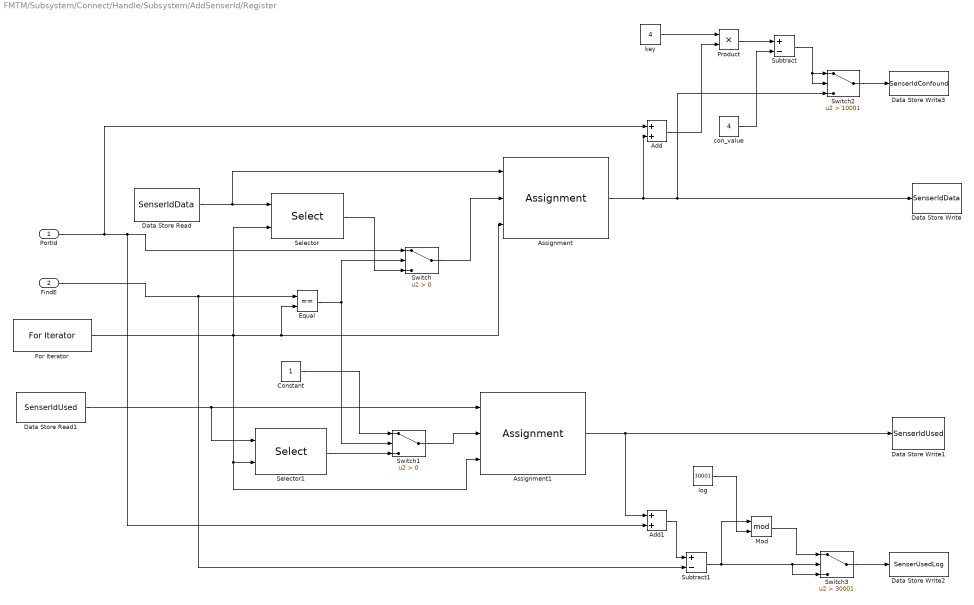
== system FMTM/Subsystem/Connect/Handle/Subsystem/AddSenserId/Register ==
  PortId : Inport
  FindE : Inport  Port=2
  Add : Sum  OutDataTypeStr=int32
  Add1 : Sum  OutDataTypeStr=int32
  Assignment : Assignment  IndexMode=Zero-based  DiagnosticForDimensions=Warning  IndexOptions=Index vector (port)  Indices=1  OutputSizes=1
  Assignment1 : Assignment  IndexMode=Zero-based  DiagnosticForDimensions=Warning  IndexOptions=Index vector (port)  Indices=1  OutputSizes=1
  Constant : Constant  OutDataTypeStr=int32
  Data Store Read : DataStoreRead  DataStoreName=SenserIdData  IndexOptions=Index vector (dialog)  Indices=1  OutputSizes=1
  Data Store Read1 : DataStoreRead  DataStoreName=SenserIdUsed  IndexOptions=Index vector (dialog)  Indices=1  OutputSizes=1
  Data Store Write : DataStoreWrite  DataStoreName=SenserIdData  IndexOptions=Index vector (dialog)  Indices=1  OutputSizes=1
  Data Store Write1 : DataStoreWrite  DataStoreName=SenserIdUsed  IndexOptions=Index vector (dialog)  Indices=1  OutputSizes=1
  Data Store Write2 : DataStoreWrite  DataStoreName=SenserUsedLog  IndexOptions=Index vector (dialog)  Indices=1  OutputSizes=1
  Data Store Write3 : DataStoreWrite  DataStoreName=SenserIdConfound  IndexOptions=Index vector (dialog)  Indices=1  OutputSizes=1
  Equal : RelationalOperator  Operator===  OutDataTypeStr=boolean  RndMeth=Simplest  InputSameDT=off
  For Iterator : ForIterator  IterationLimit=POOL_SIZE  IndexMode=Zero-based
  Mod : Math  Operator=mod
  Product : Product  OutDataTypeStr=int32
  Selector : Selector  IndexMode=Zero-based  InputPortWidth=POOL_SIZE  IndexOptions=Index vector (port)  Indices=[1 3]  OutputSizes=1
  Selector1 : Selector  IndexMode=Zero-based  InputPortWidth=POOL_SIZE  IndexOptions=Index vector (port)  Indices=[1 3]  OutputSizes=1
  Subtract : Sum  Inputs=+-  OutDataTypeStr=int32
  Subtract1 : Sum  Inputs=+-  OutDataTypeStr=int32
  Switch : Switch  Criteria=u2 > Threshold  SaturateOnIntegerOverflow=off  InputSameDT=off
  Switch1 : Switch  Criteria=u2 > Threshold  SaturateOnIntegerOverflow=off  InputSameDT=off
  Switch2 : Switch  Criteria=u2 > Threshold  Threshold=10001  SaturateOnIntegerOverflow=off  InputSameDT=off
  Switch3 : Switch  Criteria=u2 > Threshold  Threshold=30001  SaturateOnIntegerOverflow=off  InputSameDT=off
  con_value : Constant  Value=4  OutDataTypeStr=int32
  key : Constant  Value=4  OutDataTypeStr=int32
  log : Constant  Value=30001  OutDataTypeStr=int32
  wires:
  For Iterator/1 -> Assignment1/3, Selector1/2, Selector/2, Assignment/3, Equal/2
  Data Store Read/1 -> Assignment/1, Selector/1
  FindE/1 -> Subtract1/2, Equal/1
  Equal/1 -> Switch1/2, Switch/2
  PortId/1 -> Add/1, Add1/2, Switch/1
  Switch/1 -> Assignment/2
  Selector/1 -> Switch/3
  Assignment/1 -> Add/2, Switch2/3, Data Store Write/1
  Data Store Read1/1 -> Selector1/1, Assignment1/1
  Constant/1 -> Switch1/1
  Selector1/1 -> Switch1/3
  Switch1/1 -> Assignment1/2
  Assignment1/1 -> Add1/1, Data Store Write1/1
  Add/1 -> Product/2
  key/1 -> Product/1
  Product/1 -> Subtract/1
  con_value/1 -> Subtract/2
  Subtract/1 -> Switch2/2, Switch2/1
  Switch2/1 -> Data Store Write3/1
  Add1/1 -> Subtract1/1
  Subtract1/1 -> Mod/1, Switch3/3, Switch3/2
  log/1 -> Mod/2
  Mod/1 -> Switch3/1
  Switch3/1 -> Data Store Write2/1

== system FMTM/Subsystem/Disconnect/Handle/Find/Subsystem/Err ==
  Action Port : ActionPort  ActionPortLabel=if(u1 ~= 0)
  Constant : Constant  Value=-8  OutDataTypeStr=int32
  Constant1 : Constant  OutDataTypeStr=int32
  Result : Outport
  R : Outport  Port=2
  wires:
  Constant/1 -> Result/1
  Constant1/1 -> R/1

== system FMTM/Subsystem/Disconnect/Handle/Find/Subsystem/SetSenserId ==
  SenserId : Inport
  Action Port : ActionPort  ActionPortLabel=else
  Constant : Constant  OutDataTypeStr=int32
  Disconnect : Subsystem  TreatAsAtomicUnit=on
  Res : Outport
  R : Outport  Port=2
  wires:
  SenserId/1 -> Res/1, Disconnect/1(FindId)
  Constant/1 -> R/1

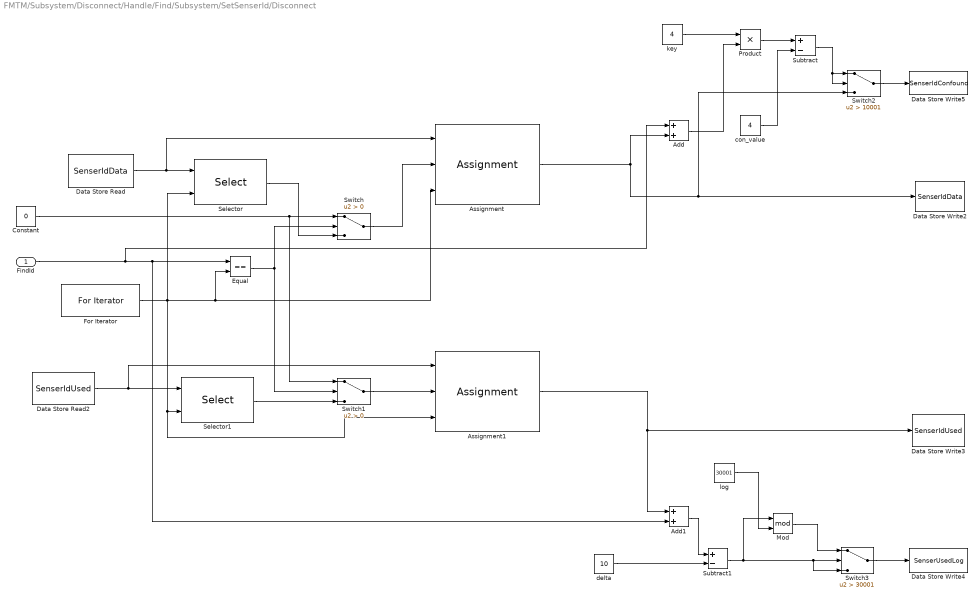
== system FMTM/Subsystem/Disconnect/Handle/Find/Subsystem/SetSenserId/Disconnect ==
  FindId : Inport
  Add : Sum  OutDataTypeStr=int32
  Add1 : Sum  OutDataTypeStr=int32
  Assignment : Assignment  IndexMode=Zero-based  DiagnosticForDimensions=Warning  IndexOptions=Index vector (port)  Indices=1  OutputSizes=1
  Assignment1 : Assignment  IndexMode=Zero-based  DiagnosticForDimensions=Warning  IndexOptions=Index vector (port)  Indices=1  OutputSizes=1
  Constant : Constant  Value=0  OutDataTypeStr=int32
  Data Store Read : DataStoreRead  DataStoreName=SenserIdData  IndexOptions=Index vector (dialog)  Indices=1  OutputSizes=1
  Data Store Read2 : DataStoreRead  DataStoreName=SenserIdUsed  IndexOptions=Index vector (dialog)  Indices=1  OutputSizes=1
  Data Store Write2 : DataStoreWrite  DataStoreName=SenserIdData  IndexOptions=Index vector (dialog)  Indices=1  OutputSizes=1
  Data Store Write3 : DataStoreWrite  DataStoreName=SenserIdUsed  IndexOptions=Index vector (dialog)  Indices=1  OutputSizes=1
  Data Store Write4 : DataStoreWrite  DataStoreName=SenserUsedLog  IndexOptions=Index vector (dialog)  Indices=1  OutputSizes=1
  Data Store Write5 : DataStoreWrite  DataStoreName=SenserIdConfound  IndexOptions=Index vector (dialog)  Indices=1  OutputSizes=1
  Equal : RelationalOperator  Operator===  OutDataTypeStr=boolean  RndMeth=Simplest  InputSameDT=off
  For Iterator : ForIterator  IterationLimit=POOL_SIZE  IndexMode=Zero-based
  Mod : Math  Operator=mod
  Product : Product  OutDataTypeStr=int32
  Selector : Selector  IndexMode=Zero-based  InputPortWidth=POOL_SIZE  IndexOptions=Index vector (port)  Indices=[1 3]  OutputSizes=1
  Selector1 : Selector  IndexMode=Zero-based  InputPortWidth=POOL_SIZE  IndexOptions=Index vector (port)  Indices=[1 3]  OutputSizes=1
  Subtract : Sum  Inputs=+-  OutDataTypeStr=int32
  Subtract1 : Sum  Inputs=+-  OutDataTypeStr=int32
  Switch : Switch  Criteria=u2 > Threshold  SaturateOnIntegerOverflow=off  InputSameDT=off
  Switch1 : Switch  Criteria=u2 > Threshold  SaturateOnIntegerOverflow=off  InputSameDT=off
  Switch2 : Switch  Criteria=u2 > Threshold  Threshold=10001  SaturateOnIntegerOverflow=off  InputSameDT=off
  Switch3 : Switch  Criteria=u2 > Threshold  Threshold=30001  SaturateOnIntegerOverflow=off  InputSameDT=off
  con_value : Constant  Value=4  OutDataTypeStr=int32
  delta : Constant  Value=10  OutDataTypeStr=int32
  key : Constant  Value=4  OutDataTypeStr=int32
  log : Constant  Value=30001  OutDataTypeStr=int32
  wires:
  For Iterator/1 -> Assignment1/3, Selector1/2, Selector/2, Assignment/3, Equal/2
  Data Store Read/1 -> Assignment/1, Selector/1
  Equal/1 -> Switch/2, Switch1/2
  Switch/1 -> Assignment/2
  Selector/1 -> Switch/3
  Constant/1 -> Switch1/1, Switch/1
  Data Store Read2/1 -> Assignment1/1, Selector1/1
  Selector1/1 -> Switch1/3
  Switch1/1 -> Assignment1/2
  Switch2/1 -> Data Store Write5/1
  Subtract/1 -> Switch2/2, Switch2/1
  Switch3/1 -> Data Store Write4/1
  Subtract1/1 -> Mod/1, Switch3/3, Switch3/2
  log/1 -> Mod/2
  Product/1 -> Subtract/1
  key/1 -> Product/1
  con_value/1 -> Subtract/2
  FindId/1 -> Add/1, Add1/2, Equal/1
  Mod/1 -> Switch3/1
  Add/1 -> Product/2
  Assignment1/1 -> Add1/1, Data Store Write3/1
  Assignment/1 -> Switch2/3, Data Store Write2/1, Add/2
  Add1/1 -> Subtract1/1
  delta/1 -> Subtract1/2
